simulink model "OFDM"  (R2016b)
settings: Solver=VariableStepAuto  StartTime=0.0  StopTime=10/300  RelTol=1e-3
libraries: dsparch4 x7, commsrccod2 x2, commutil2 x2, commchan3 x1, commsink2 x1, commnoisgen2 x1
settings Model: Creator=white  LastModifiedBy=white

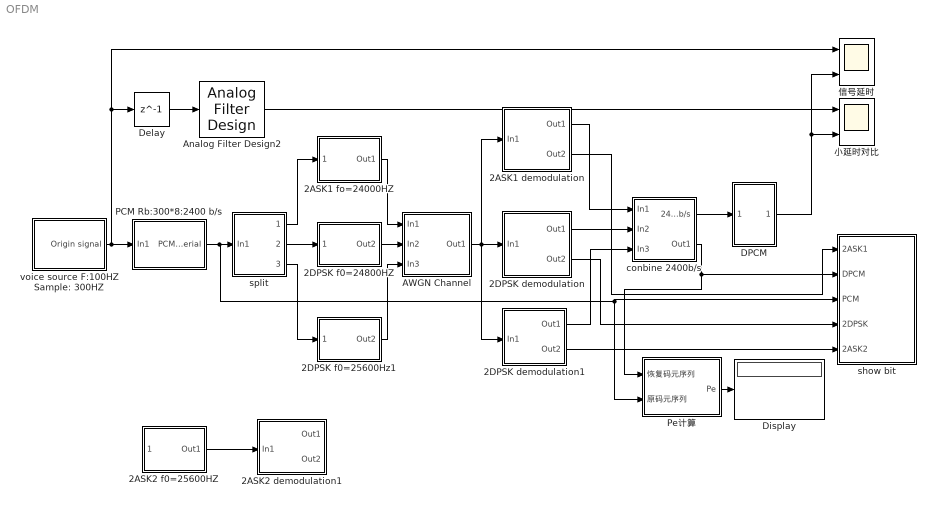
== system OFDM ==
  2ASK1 fo=24000HZ : Subsystem
  2ASK1 demodulation : Subsystem
  2ASK2 f0=25600HZ : Subsystem
  2ASK2 demodulation1 : Subsystem
  2DPSK f0=24800HZ : Subsystem
  2DPSK f0=25600Hz1 : Subsystem
  2DPSK demodulation : Subsystem
  2DPSK demodulation1 : Subsystem
  AWGN Channel : Subsystem
  Analog Filter Design2 : dsparch4/Analog Filter Design  method=Butterworth  filttype=Lowpass  N=7  Wlo=2*100*pi  Whi=80  Rp=2  Rs=40
  "DPCM " : Subsystem
  Delay : Delay  DelayLength=1  InitialCondition=0  SampleTime=1/300
  Display : Display
  PCM Rb:300*8:2400 b/s : Subsystem
  Pe计算 : Subsystem
  conbine 2400b/s : Subsystem
  show bit : Subsystem
  split : Subsystem
  voice source F:100HZ Sample: 300HZ : Subsystem
  信号延时 : Scope  NumInputPorts=2
  小延时对比 : Scope  NumInputPorts=2
  wires:
  PCM Rb:300*8:2400 b/s/1(PCM Serial) -> Pe计算/2(原码元序列), show bit/3(PCM), split/1(In1)
  split/1(2ASK1) -> 2ASK1 fo=24000HZ/1(800b/s)
  split/2(2DPSK) -> 2DPSK f0=24800HZ/1(800b/s)
  2ASK1 fo=24000HZ/1(Out1) -> AWGN Channel/1(In1)
  2DPSK f0=24800HZ/1(Out2) -> AWGN Channel/2(In2)
  2DPSK f0=25600Hz1/1(Out2) -> AWGN Channel/3(In3)
  AWGN Channel/1(Out1) -> 2DPSK demodulation1/1(In1), 2DPSK demodulation/1(In1), 2ASK1 demodulation/1(In1)
  2ASK1 demodulation/1(Out1) -> conbine 2400b/s/1(In1)
  2DPSK demodulation/1(Out1) -> conbine 2400b/s/2(In2)
  2DPSK demodulation1/1(Out1) -> conbine 2400b/s/3(In3)
  conbine 2400b/s/1(2400b/s) -> "DPCM "/1(In1)
  2ASK1 demodulation/2(Out2) -> show bit/1(2ASK1)
  conbine 2400b/s/2(Out1) -> Pe计算/1(恢复码元序列), show bit/2(DPCM)
  2DPSK demodulation/2(Out2) -> show bit/4(2DPSK)
  voice source F:100HZ Sample: 300HZ/1(Origin signal) -> PCM Rb:300*8:2400 b/s/1(In1), 信号延时/1, Delay/1
  Delay/1 -> Analog Filter Design2/1
  split/3(2ASK2) -> 2DPSK f0=25600Hz1/1(800b/s)
  Pe计算/1(Pe) -> Display/1
  "DPCM "/1(Out1) -> 小延时对比/2, 信号延时/2
  Analog Filter Design2/1 -> 小延时对比/1
  2DPSK demodulation1/2(Out2) -> show bit/5(2ASK2)
  2ASK2 f0=25600HZ/1(Out1) -> 2ASK2 demodulation1/1(In1)

== system OFDM/2ASK1 fo=24000HZ ==
  800b/s : Inport
  Product : Product
  Sine Wave : Sin  Frequency=24000*2*pi  SampleTime=0
  Out1 : Outport
  wires:
  800b/s/1 -> Product/2
  Sine Wave/1 -> Product/1
  Product/1 -> Out1/1

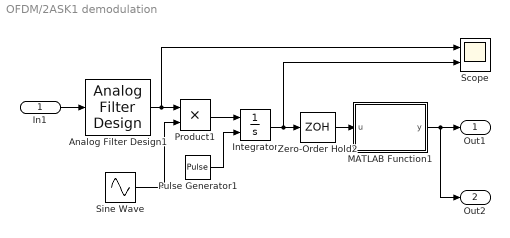
== system OFDM/2ASK1 demodulation ==
  In1 : Inport
  Analog Filter Design1 : dsparch4/Analog Filter Design  method=Butterworth  filttype=Bandpass  N=1  Wlo=2*23200*pi  Whi=2*24800*pi  Rp=2  Rs=40
  Integrator : Integrator  ExternalReset=rising
  MATLAB Function1 : MATLAB Function  TreatAsAtomicUnit=on
  Product1 : Product
  Pulse Generator1 : DiscretePulseGenerator  PulseType=Time based  Period=1/800  PulseWidth=5  PhaseDelay=1/8000
  Scope : Scope  NumInputPorts=2
  Sine Wave : Sin  Frequency=24000*2*pi  SampleTime=0
  Zero-Order Hold2 : ZeroOrderHold  SampleTime=1/800
  Out1 : Outport
  Out2 : Outport  Port=2
  wires:
  Analog Filter Design1/1 -> Scope/1, Product1/1
  Product1/1 -> Integrator/1
  Pulse Generator1/1 -> Integrator/2
  Integrator/1 -> Scope/2, Zero-Order Hold2/1
  In1/1 -> Analog Filter Design1/1
  Sine Wave/1 -> Product1/2
  MATLAB Function1/1(y) -> Out2/1, Out1/1
  Zero-Order Hold2/1 -> MATLAB Function1/1(u)

== system OFDM/2ASK2 f0=25600HZ ==
  800b/s : Inport
  Product : Product
  Sine Wave : Sin  Frequency=25600*2*pi  SampleTime=0
  Out1 : Outport
  wires:
  800b/s/1 -> Product/2
  Sine Wave/1 -> Product/1
  Product/1 -> Out1/1

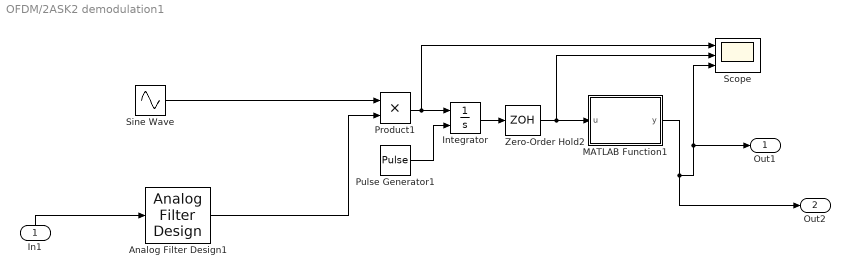
== system OFDM/2ASK2 demodulation1 ==
  In1 : Inport
  Analog Filter Design1 : dsparch4/Analog Filter Design  method=Butterworth  filttype=Bandpass  N=1  Wlo=2*24800*pi  Whi=2*26200*pi  Rp=2  Rs=40
  Integrator : Integrator  ExternalReset=rising
  MATLAB Function1 : MATLAB Function  TreatAsAtomicUnit=on
  Product1 : Product
  Pulse Generator1 : DiscretePulseGenerator  PulseType=Time based  Period=1/800  PulseWidth=5  PhaseDelay=1/8000  VectorParams1D=off
  Scope : Scope  NumInputPorts=3
  Sine Wave : Sin  Frequency=25600*2*pi  SampleTime=0
  Zero-Order Hold2 : ZeroOrderHold  SampleTime=1/800
  Out1 : Outport
  Out2 : Outport  Port=2
  wires:
  Product1/1 -> Scope/1, Integrator/1
  Pulse Generator1/1 -> Integrator/2
  Integrator/1 -> Zero-Order Hold2/1
  In1/1 -> Analog Filter Design1/1
  Zero-Order Hold2/1 -> MATLAB Function1/1(u), Scope/2
  MATLAB Function1/1(y) -> Scope/3, Out1/1, Out2/1
  Analog Filter Design1/1 -> Product1/2
  Sine Wave/1 -> Product1/1

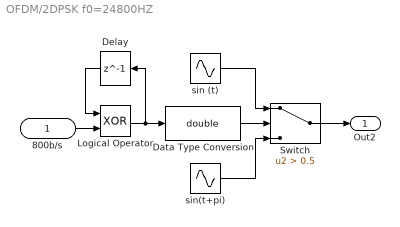
== system OFDM/2DPSK f0=24800HZ ==
  800b/s : Inport
  Data Type Conversion : DataTypeConversion  OutDataTypeStr=double
  Delay : Delay  DelayLength=1  InitialCondition=0  SampleTime=1/800
  Logical Operator : Logic  Operator=XOR  AllPortsSameDT=off  OutDataTypeStr=boolean
  Switch : Switch  Criteria=u2 > Threshold  Threshold=0.5
  sin (t) : Sin  Frequency=2*24800*pi  SampleTime=0
  sin(t+pi) : Sin  Frequency=2*pi*24800  Phase=pi  SampleTime=0
  Out2 : Outport
  wires:
  sin (t)/1 -> Switch/1
  Switch/1 -> Out2/1
  Logical Operator/1 -> Data Type Conversion/1, Delay/1
  Data Type Conversion/1 -> Switch/2
  sin(t+pi)/1 -> Switch/3
  800b/s/1 -> Logical Operator/2
  Delay/1 -> Logical Operator/1

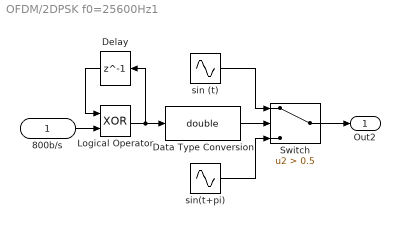
== system OFDM/2DPSK f0=25600Hz1 ==
  800b/s : Inport
  Data Type Conversion : DataTypeConversion  OutDataTypeStr=double
  Delay : Delay  DelayLength=1  InitialCondition=0  SampleTime=1/800
  Logical Operator : Logic  Operator=XOR  AllPortsSameDT=off  OutDataTypeStr=boolean
  Switch : Switch  Criteria=u2 > Threshold  Threshold=0.5
  sin (t) : Sin  Frequency=2*25600*pi  SampleTime=0
  sin(t+pi) : Sin  Frequency=2*pi*25600  Phase=pi  SampleTime=0
  Out2 : Outport
  wires:
  Delay/1 -> Logical Operator/1
  800b/s/1 -> Logical Operator/2
  sin(t+pi)/1 -> Switch/3
  Data Type Conversion/1 -> Switch/2
  Logical Operator/1 -> Delay/1, Data Type Conversion/1
  Switch/1 -> Out2/1
  sin (t)/1 -> Switch/1

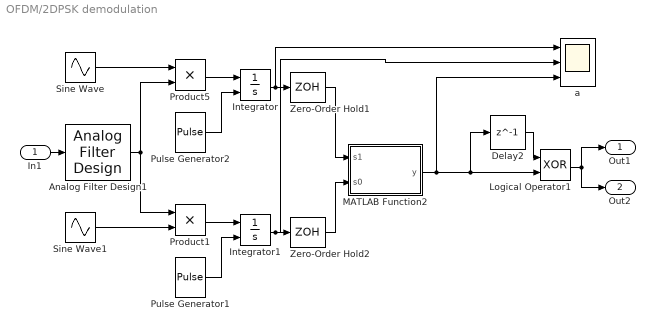
== system OFDM/2DPSK demodulation ==
  In1 : Inport
  Analog Filter Design1 : dsparch4/Analog Filter Design  method=Butterworth  filttype=Bandpass  N=1  Wlo=2*24000*pi  Whi=2*25600*pi  Rp=2  Rs=40
  Delay2 : Delay  DelayLength=1  InitialCondition=0  SampleTime=1/800
  Integrator : Integrator  ExternalReset=rising
  Integrator1 : Integrator  ExternalReset=rising
  Logical Operator1 : Logic  Operator=XOR  AllPortsSameDT=off  OutDataTypeStr=boolean
  MATLAB Function2 : MATLAB Function  TreatAsAtomicUnit=on
  Product1 : Product
  Product5 : Product
  Pulse Generator1 : DiscretePulseGenerator  PulseType=Time based  Period=1/800  PulseWidth=5  PhaseDelay=1/8000
  Pulse Generator2 : DiscretePulseGenerator  PulseType=Time based  Period=1/800  PulseWidth=5  PhaseDelay=1/8000
  Sine Wave : Sin  Frequency=2*24800*pi  SampleTime=0
  Sine Wave1 : Sin  Frequency=2*24800*pi  Phase=pi  SampleTime=0
  Zero-Order Hold1 : ZeroOrderHold  SampleTime=1/800
  Zero-Order Hold2 : ZeroOrderHold  SampleTime=1/800
  a : Scope  NumInputPorts=3
  Out1 : Outport
  Out2 : Outport  Port=2
  wires:
  MATLAB Function2/1(y) -> a/3, Logical Operator1/2, Delay2/1
  Sine Wave/1 -> Product5/1
  Pulse Generator2/1 -> Integrator/2
  Product5/1 -> Integrator/1
  Integrator/1 -> a/1, Zero-Order Hold1/1
  Analog Filter Design1/1 -> Product5/2, Product1/1
  In1/1 -> Analog Filter Design1/1
  Logical Operator1/1 -> Out2/1, Out1/1
  Zero-Order Hold1/1 -> MATLAB Function2/1(s1)
  Pulse Generator1/1 -> Integrator1/2
  Product1/1 -> Integrator1/1
  Integrator1/1 -> a/2, Zero-Order Hold2/1
  Sine Wave1/1 -> Product1/2
  Zero-Order Hold2/1 -> MATLAB Function2/2(s0)
  Delay2/1 -> Logical Operator1/1

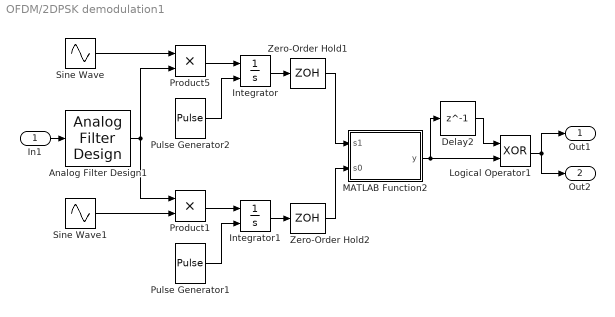
== system OFDM/2DPSK demodulation1 ==
  In1 : Inport
  Analog Filter Design1 : dsparch4/Analog Filter Design  method=Butterworth  filttype=Bandpass  N=1  Wlo=2*24800*pi  Whi=2*26200*pi  Rp=2  Rs=40
  Delay2 : Delay  DelayLength=1  InitialCondition=0  SampleTime=1/800
  Integrator : Integrator  ExternalReset=rising
  Integrator1 : Integrator  ExternalReset=rising
  Logical Operator1 : Logic  Operator=XOR  AllPortsSameDT=off  OutDataTypeStr=boolean
  MATLAB Function2 : MATLAB Function  TreatAsAtomicUnit=on
  Product1 : Product
  Product5 : Product
  Pulse Generator1 : DiscretePulseGenerator  PulseType=Time based  Period=1/800  PulseWidth=5  PhaseDelay=1/8000
  Pulse Generator2 : DiscretePulseGenerator  PulseType=Time based  Period=1/800  PulseWidth=5  PhaseDelay=1/8000
  Sine Wave : Sin  Frequency=2*25600*pi  SampleTime=0
  Sine Wave1 : Sin  Frequency=2*25600*pi  Phase=pi  SampleTime=0
  Zero-Order Hold1 : ZeroOrderHold  SampleTime=1/800
  Zero-Order Hold2 : ZeroOrderHold  SampleTime=1/800
  Out1 : Outport
  Out2 : Outport  Port=2
  wires:
  Delay2/1 -> Logical Operator1/1
  Zero-Order Hold2/1 -> MATLAB Function2/2(s0)
  Sine Wave1/1 -> Product1/2
  Integrator1/1 -> Zero-Order Hold2/1
  Product1/1 -> Integrator1/1
  Pulse Generator1/1 -> Integrator1/2
  Zero-Order Hold1/1 -> MATLAB Function2/1(s1)
  Logical Operator1/1 -> Out1/1, Out2/1
  In1/1 -> Analog Filter Design1/1
  Analog Filter Design1/1 -> Product1/1, Product5/2
  Integrator/1 -> Zero-Order Hold1/1
  Product5/1 -> Integrator/1
  Pulse Generator2/1 -> Integrator/2
  Sine Wave/1 -> Product5/1
  MATLAB Function2/1(y) -> Delay2/1, Logical Operator1/2

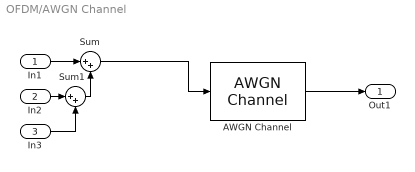
== system OFDM/AWGN Channel ==
  In1 : Inport
  In2 : Inport  Port=2
  In3 : Inport  Port=3
  AWGN Channel : commchan3/AWGN Channel  InputProcessing=Columns as channels (frame based)  seed=67  noiseMode=Variance from mask  EbNodB=10  EsNodB=10  SNRdB=10  bitsPerSym=800  Ps=1  Tsym=1  variance=0.005
  Sum : Sum  Inputs=|++
  Sum1 : Sum  Inputs=|++
  Out1 : Outport
  wires:
  In1/1 -> Sum/1
  Sum1/1 -> Sum/2
  Sum/1 -> AWGN Channel/1
  In2/1 -> Sum1/1
  In3/1 -> Sum1/2
  AWGN Channel/1 -> Out1/1

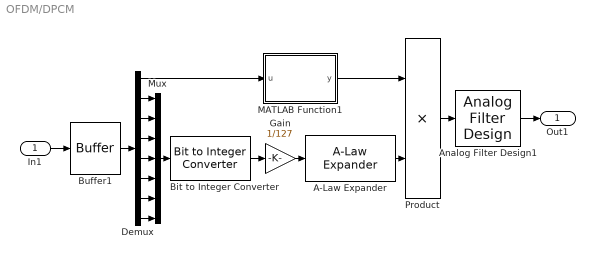
== system OFDM/DPCM  ==
  In1 : Inport
  A-Law Expander : commsrccod2/A-Law Expander  A=87.6  V=1
  Analog Filter Design1 : dsparch4/Analog Filter Design  method=Butterworth  filttype=Lowpass  N=7  Wlo=2*100*pi  Whi=80  Rp=2  Rs=40
  Bit to Integer Converter : commutil2/Bit to Integer Converter  nbits=7  bitOrder=MSB first  signedOutputValues=Unsigned  outDtype=Inherit via internal rule  outDtypeSigned=Inherit via internal rule
  Buffer1 : Buffer  N=8  TreatMby1Signals=One channel  OutputFrames=off
  Demux : Demux  Outputs=8
  Gain : Gain  Gain=1/127
  MATLAB Function1 : MATLAB Function  TreatAsAtomicUnit=on
  Mux : Mux  Inputs=7
  Product : Product
  Out1 : Outport
  wires:
  Demux/2 -> Mux/1
  Demux/3 -> Mux/2
  Demux/4 -> Mux/3
  Demux/5 -> Mux/4
  Demux/6 -> Mux/5
  Demux/7 -> Mux/6
  Demux/8 -> Mux/7
  Bit to Integer Converter/1 -> Gain/1
  Mux/1 -> Bit to Integer Converter/1
  Gain/1 -> A-Law Expander/1
  Demux/1 -> MATLAB Function1/1(u)
  A-Law Expander/1 -> Product/2
  Buffer1/1 -> Demux/1
  Product/1 -> Analog Filter Design1/1
  Analog Filter Design1/1 -> Out1/1
  In1/1 -> Buffer1/1
  MATLAB Function1/1(y) -> Product/1

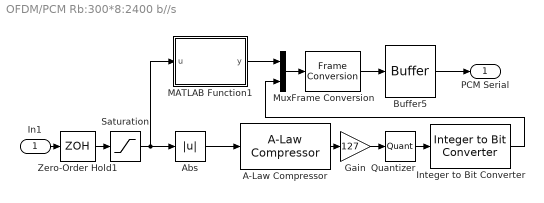
== system OFDM/PCM Rb:300*8:2400 b//s ==
  In1 : Inport
  A-Law Compressor : commsrccod2/A-Law Compressor  A=87.6  V=1
  Abs : Abs
  Buffer5 : Buffer  N=1  TreatMby1Signals=One channel  OutputFrames=off
  Frame Conversion : FrameConversion  InheritSamplingMode=off
  Gain : Gain  Gain=127
  Integer to Bit Converter : commutil2/Integer to Bit Converter  nbits=7  signedInputValues=Unsigned  bitOrder=MSB first  outDtype=Inherit via internal rule
  MATLAB Function1 : MATLAB Function  TreatAsAtomicUnit=on
  Mux : Mux  Inputs=2
  Quantizer : Quantizer  QuantizationInterval=1
  Saturation : Saturate  UpperLimit=1  LowerLimit=-1
  Zero-Order Hold1 : ZeroOrderHold  SampleTime=1/300
  PCM Serial : Outport
  wires:
  In1/1 -> Zero-Order Hold1/1
  Abs/1 -> A-Law Compressor/1
  A-Law Compressor/1 -> Gain/1
  Integer to Bit Converter/1 -> Mux/2
  Gain/1 -> Quantizer/1
  Quantizer/1 -> Integer to Bit Converter/1
  Saturation/1 -> MATLAB Function1/1(u), Abs/1
  Mux/1 -> Frame Conversion/1
  Zero-Order Hold1/1 -> Saturation/1
  Frame Conversion/1 -> Buffer5/1
  Buffer5/1 -> PCM Serial/1
  MATLAB Function1/1(y) -> Mux/1

== system OFDM/Pe计算 ==
  恢复码元序列 : Inport
  原码元序列 : Inport  Port=2
  Data Type Conversion : DataTypeConversion  OutDataTypeStr=double
  Data Type Conversion1 : DataTypeConversion  OutDataTypeStr=double
  Error Rate Calculation : commsink2/Error Rate Calculation  N=6  st_delay=0  cp_mode=Entire frame  subframe=[]  PMode=Port  WsName=ErrorVec  RsMode2=off  stop=off  numErr=100  maxBits=1e6
  Pe : Outport
  wires:
  原码元序列/1 -> Data Type Conversion/1
  恢复码元序列/1 -> Data Type Conversion1/1
  Data Type Conversion/1 -> Error Rate Calculation/1
  Error Rate Calculation/1 -> Pe/1
  Data Type Conversion1/1 -> Error Rate Calculation/2

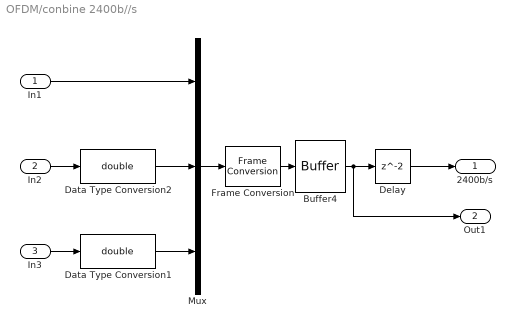
== system OFDM/conbine 2400b//s ==
  In1 : Inport
  In2 : Inport  Port=2
  In3 : Inport  Port=3
  Buffer4 : Buffer  N=1  TreatMby1Signals=One channel  OutputFrames=off
  Data Type Conversion1 : DataTypeConversion  OutDataTypeStr=double
  Data Type Conversion2 : DataTypeConversion  OutDataTypeStr=double
  Delay : Delay  InitialCondition=0  SampleTime=1/2400
  Frame Conversion : FrameConversion  InheritSamplingMode=off
  Mux : Mux  Inputs=3
  2400b/s : Outport
  Out1 : Outport  Port=2
  wires:
  In1/1 -> Mux/1
  In3/1 -> Data Type Conversion1/1
  In2/1 -> Data Type Conversion2/1
  Delay/1 -> 2400b/s/1
  Buffer4/1 -> Out1/1, Delay/1
  Mux/1 -> Frame Conversion/1
  Frame Conversion/1 -> Buffer4/1
  Data Type Conversion2/1 -> Mux/2
  Data Type Conversion1/1 -> Mux/3

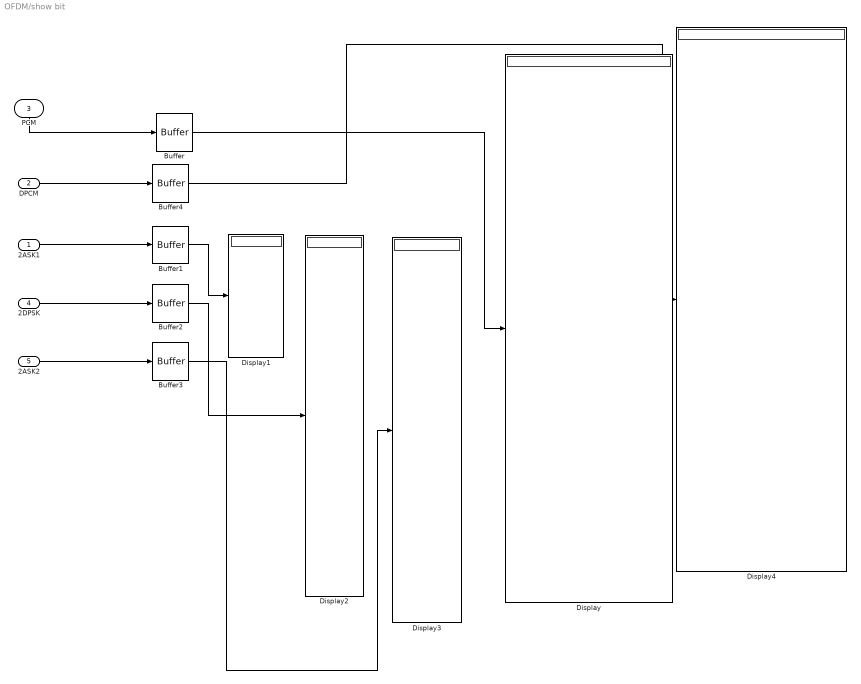
== system OFDM/show bit ==
  2ASK1 : Inport
  DPCM : Inport  Port=2
  PCM : Inport  Port=3
  2DPSK : Inport  Port=4
  2ASK2 : Inport  Port=5
  Buffer : Buffer  N=15*8  TreatMby1Signals=One channel  OutputFrames=off
  Buffer1 : Buffer  N=8  TreatMby1Signals=One channel  OutputFrames=off
  Buffer2 : Buffer  N=8  TreatMby1Signals=One channel  OutputFrames=off
  Buffer3 : Buffer  N=8  TreatMby1Signals=One channel  OutputFrames=off
  Buffer4 : Buffer  N=15*8  TreatMby1Signals=One channel  OutputFrames=off
  Display{,1..4} (5 alike) : Display
  wires:
  PCM/1 -> Buffer/1
  Buffer/1 -> Display/1
  Buffer4/1 -> Display4/1
  2DPSK/1 -> Buffer2/1
  2ASK2/1 -> Buffer3/1
  Buffer1/1 -> Display1/1
  Buffer3/1 -> Display3/1
  Buffer2/1 -> Display2/1
  2ASK1/1 -> Buffer1/1
  DPCM/1 -> Buffer4/1

== system OFDM/split ==
  In1 : Inport
  A1 : Scope  NumInputPorts=3
  Buffer : Buffer  N=3  TreatMby1Signals=One channel  OutputFrames=off
  Demux : Demux  Outputs=3
  2ASK1 : Outport
  2DPSK : Outport  Port=2
  2ASK2 : Outport  Port=3
  wires:
  Demux/2 -> A1/2, 2DPSK/1
  Demux/3 -> 2ASK2/1, A1/3
  In1/1 -> Buffer/1
  Demux/1 -> A1/1, 2ASK1/1
  Buffer/1 -> Demux/1

== system OFDM/voice source F:100HZ Sample: 300HZ ==
  Analog Filter Design2 : dsparch4/Analog Filter Design  method=Butterworth  filttype=Lowpass  N=7  Wlo=2*100*pi  Whi=80  Rp=2  Rs=40
  Gaussian Noise Generator : commnoisgen2/Gaussian Noise Generator  m=0  d=0.3  s=41  Ts=1/100  frameBased=off  sampPerFrame=1  orient=off  outDataType=double
  Origin signal : Outport
  wires:
  Gaussian Noise Generator/1 -> Analog Filter Design2/1
  Analog Filter Design2/1 -> Origin signal/1

== matlab function OFDM/2ASK1 demodulation/MATLAB Function1 ==
  data: u input; y output
function y = fcn(u)
if(u>0.000205)
    u=1
else
    u=0
end
y = u;

== matlab function OFDM/2ASK2 demodulation1/MATLAB Function1 ==
  data: u input; y output
function y = fcn(u)
if(u>0.000205)
    u=1
else
    u=0
end
y = u;

== matlab function OFDM/PCM Rb:300*8:2400 b//s/MATLAB Function1 ==
  data: u input; y output
function y = fcn(u)
if(u>=0)
    u=0
else
    u=1
end
y = u;

== matlab function OFDM/2DPSK demodulation/MATLAB Function2 ==
  data: s1 input; y output; s0 input
function y = fcn(s1,s0)
if(s1>=s0)
    u=1
else
    u=0
end
y = u;

== matlab function OFDM/DPCM /MATLAB Function1 ==
  data: u input; y output
function y = fcn(u)
if(u>0)
    u=-1
else
    u=1
end
y = u;

== matlab function OFDM/2DPSK demodulation1/MATLAB Function2 ==
  data: s1 input; y output; s0 input
function y = fcn(s1,s0)
if(s1>=s0)
    u=1
else
    u=0
end
y = u;
